simulink model "DSB"  (R2020b)
settings: Solver=VariableStepAuto  StartTime=0.0  StopTime=0.05  RelTol=1e-3
libraries: dspsrcs4 x2, dsparch4 x1
settings Model: Creator=tamim  LastModifiedBy=Safir
settings DebuggingCC: SFMachineParentedDataDiag=error

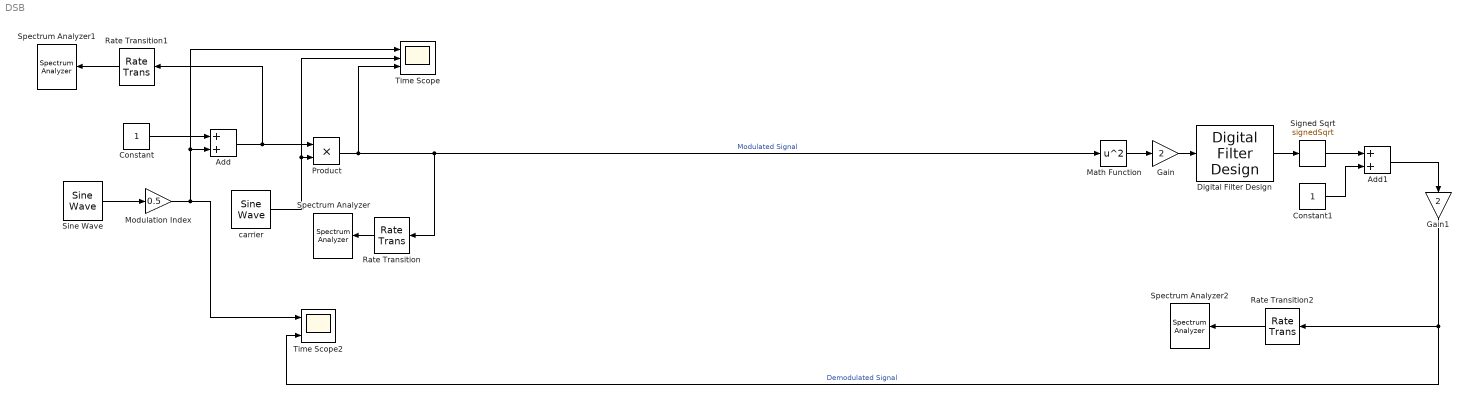
== system DSB ==
  Add : Sum
  Add1 : Sum
  Constant : Constant
  Constant1 : Constant
  Digital Filter Design : dsparch4/Digital Filter Design  mwdsp_browser_bugfix_var=off
  Gain : Gain  Gain=2
  Gain1 : Gain  Gain=2
  Math Function : Math  Operator=square  SaturateOnIntegerOverflow=on
  Modulation Index : Gain  Gain=0.5
  Product : Product
  Rate Transition : RateTransition
  Rate Transition1 : RateTransition
  Rate Transition2 : RateTransition
  Signed Sqrt : Sqrt  Operator=signedSqrt  SaturateOnIntegerOverflow=on
  Sine Wave : dspsrcs4/Sine Wave  Amplitude=1  Frequency=1000  Phase=0  SampleMode=Discrete  OutComplex=Real  CompMethod=Trigonometric fcn  TableSize=Speed  SampleTime=1/96000  SamplesPerFrame=64  ResetState=Restart at time zero  OutputFrames=off  dataType=double  wordLen=16  udDataType=sfix(16)  fracBitsMode=Best precision  numFracBits=15  OutDataTypeStr=double  LastOutDataTypeStr=double
  Spectrum Analyzer : SpectrumAnalyzer
  Spectrum Analyzer1 : SpectrumAnalyzer
  Spectrum Analyzer2 : SpectrumAnalyzer
  Time Scope : Scope  NumInputPorts=3
  Time Scope2 : Scope  NumInputPorts=2
  carrier : dspsrcs4/Sine Wave  Amplitude=1  Frequency=20000  Phase=0  SampleMode=Discrete  OutComplex=Real  CompMethod=Trigonometric fcn  TableSize=Speed  SampleTime=1/96000  SamplesPerFrame=64  ResetState=Restart at time zero  OutputFrames=off  dataType=double  wordLen=16  udDataType=sfix(16)  fracBitsMode=Best precision  numFracBits=15  OutDataTypeStr=double  LastOutDataTypeStr=double
  wires:
  Sine Wave/1 -> Modulation Index/1
  Modulation Index/1 -> Time Scope2/1, Time Scope/1, Add/2
  Constant/1 -> Add/1
  Add/1 -> Rate Transition1/1, Product/1
  carrier/1 -> Time Scope/2, Product/2
  Product/1 -> Math Function/1, Rate Transition/1, Time Scope/3  "Modulated Signal"
  Rate Transition/1 -> Spectrum Analyzer/1
  Rate Transition1/1 -> Spectrum Analyzer1/1
  Math Function/1 -> Gain/1
  Signed Sqrt/1 -> Add1/1
  Constant1/1 -> Add1/2
  Add1/1 -> Gain1/1
  Rate Transition2/1 -> Spectrum Analyzer2/1
  Gain1/1 -> Time Scope2/2, Rate Transition2/1  "Demodulated Signal"
  Gain/1 -> Digital Filter Design/1
  Digital Filter Design/1 -> Signed Sqrt/1
